simulink model "S2Z_1_Sim"  (R2025b)
settings: Solver=VariableStepAuto  StartTime=0.0  StopTime=10  RelTol=1e-3
values from neighbouring files (symbols this model uses):
  Ts = 1/Fs    (= 0.001)    [S2Z_1_.m]
undefined symbols (not defined in the file or in its folder): dspblkCoreblockFVToolHelper, gcbh, Gd, Gn, Gzd, Gzn
settings Model: LastModifiedBy=maxvega

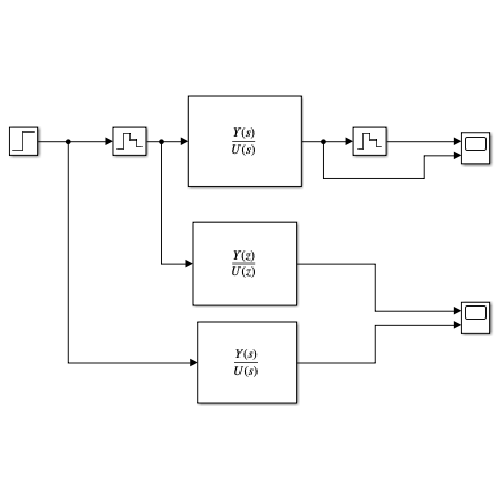
[thumbnail: Simulink's stored preview of the top-level diagram]
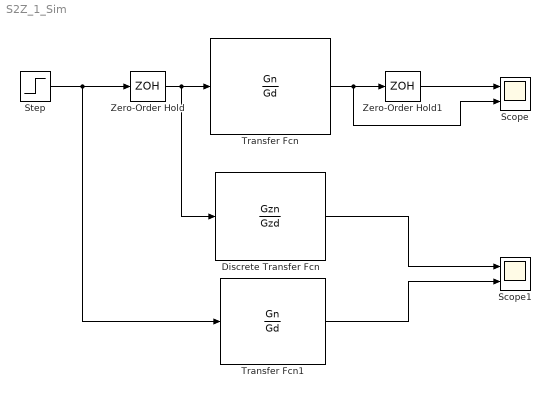
== system S2Z_1_Sim ==
  Discrete Transfer Fcn : DiscreteTransferFcn  LoadFcn=dspblkCoreblockFVToolHelper(gcbh,'load');  Numerator=Gzn  Denominator=Gzd
      settings: CopyFcn=dspblkCoreblockFVToolHelper(gcbh,'copy');  DeleteFcn=dspblkCoreblockFVToolHelper(gcbh,'close');  ModelCloseFcn=dspblkCoreblockFVToolHelper(gcbh,'close');  PreSaveFcn=dspblkCoreblockFVToolHelper(gcbh,'presave');  PostSaveFcn=dspblkCoreblockFVToolHelper(gcbh,'postsave');  CloseFcn=dspblkCoreblockFVToolHelper(gcbh,'close');
  Scope : Scope  NumInputPorts=2
      settings: ActiveDisplayYMinimum=0.17796389552320935  ActiveDisplayYMaximum=0.17817233841643876
  Scope1 : Scope  NumInputPorts=2
      settings: ActiveDisplayYMinimum=0.26881276884758049  ActiveDisplayYMaximum=0.31048469094499692
  Step : Step  Time=0  SampleTime=0
  Transfer Fcn : TransferFcn  Numerator=Gn  Denominator=Gd
  Transfer Fcn1 : TransferFcn  Numerator=Gn  Denominator=Gd
  Zero-Order Hold : ZeroOrderHold  SampleTime=Ts
  Zero-Order Hold1 : ZeroOrderHold  SampleTime=Ts
  wires:
  Step/1 -> Transfer Fcn1/1, Zero-Order Hold/1
  Zero-Order Hold/1 -> Discrete Transfer Fcn/1, Transfer Fcn/1
  Transfer Fcn/1 -> Scope/2, Zero-Order Hold1/1
  Zero-Order Hold1/1 -> Scope/1
  Discrete Transfer Fcn/1 -> Scope1/1
  Transfer Fcn1/1 -> Scope1/2
